simulink model "cardiac_dynamic_model"  (R2019b)
settings: Solver=FixedStepAuto  StartTime=0.0  StopTime=1  FixedStep=1e-4  RelTol=1e-3
settings Model: Creator=User  LastModifiedBy=User

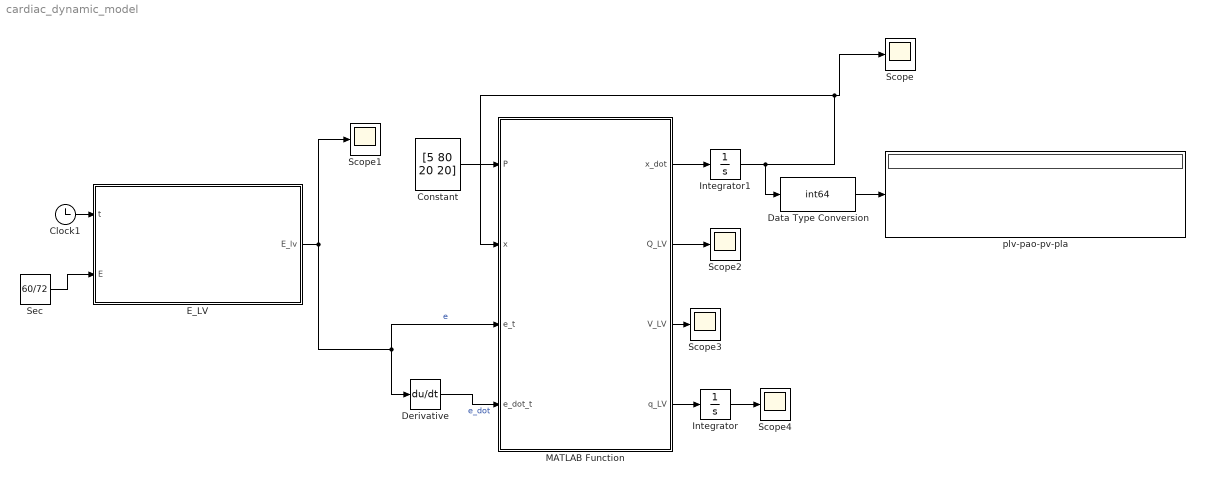
== system cardiac_dynamic_model ==
  Clock1 : Clock
  Constant : Constant  Value=[5 80 20 20]
  Data Type Conversion : DataTypeConversion  OutDataTypeStr=int64  RndMeth=Round
  Derivative : Derivative
  E_LV : Subsystem
  Integrator : Integrator
  Integrator1 : Integrator
  MATLAB Function : MATLAB Function  TreatAsAtomicUnit=on
  Scope{,1..4} (5 alike) : Scope
  Sec : Constant  Value=60/72
  plv-pao-pv-pla : Display
  wires:
  E_LV/1(E_lv) -> MATLAB Function/3(e_t), Derivative/1, Scope1/1  "e"
  Derivative/1 -> MATLAB Function/4(e_dot_t)  "e_dot"
  MATLAB Function/4(q_LV) -> Integrator/1
  MATLAB Function/2(Q_LV) -> Scope2/1
  MATLAB Function/3(V_LV) -> Scope3/1
  Integrator/1 -> Scope4/1
  Clock1/1 -> E_LV/1(t)
  Sec/1 -> E_LV/2(E)
  Integrator1/1 -> Data Type Conversion/1, MATLAB Function/2(x), Scope/1
  Data Type Conversion/1 -> plv-pao-pv-pla/1
  Constant/1 -> MATLAB Function/1(P)
  MATLAB Function/1(x_dot) -> Integrator1/1

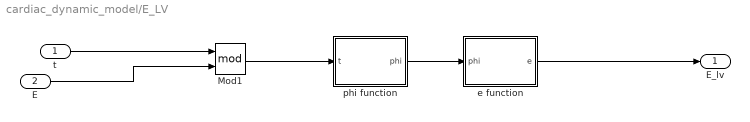
== system cardiac_dynamic_model/E_LV ==
  t : Inport
  E : Inport  Port=2
  Mod1 : Math  Operator=mod  SignedPower=off  SaturateOnIntegerOverflow=on
  e function : MATLAB Function  TreatAsAtomicUnit=on
  phi function : MATLAB Function  TreatAsAtomicUnit=on
  E_lv : Outport
  wires:
  e function/1(e) -> E_lv/1
  phi function/1(phi) -> e function/1(phi)
  Mod1/1 -> phi function/1(t)
  t/1 -> Mod1/1
  E/1 -> Mod1/2

== matlab function cardiac_dynamic_model/E_LV/phi function ==
  data: t input; phi output
function phi = fcn(t)
phi = 0.9*sin(pi/0.4*t)-0.25*sin(2*pi/0.4*t);
end

== matlab function cardiac_dynamic_model/MATLAB Function ==
  data: P input; x input; x_dot output; e_t input; e_dot_t input; Q_LV output; V_LV output; q_LV output
function [x_dot,Q_LV, V_LV, q_LV] = cardiovascular_model(P,x,e_t,e_dot_t)
Q = zeros(2,1);
p1 = 0; p2 = 0;
G1= 14.81; G2=1.46; G3=266.6; G4=20;
E_1=1/0.22;  E_2=1/20; E_3=1/1.46; E_4=1/200;
P1=5; P2=80; P3=20; P4=20;
if ((P4 - P1) > 0)
    p1 = P4 - P1;
end
    if ((P1 - P2)> 0)
        p2 = P1 - P2;
    end
    Q = [G3*p1; G2*p2];
    phase = 0;
    if Q(2,1) > 0 && Q(1,1) == 0
        phase = 1;
        G3=0;
    end
    if Q(1,1) > 0 && Q(2,1) == 0
        phase = 2;
        G2=0;
    end
    A= [e_dot_t.*4*E_4-(G3+G1) E_4/G1 0 E_4/G3;
       E_1*G2 -E_1*(G2+G1) E_1*G1 0;
     0 E_2*G1 -E_2*(G1+G4) E_2*G4;
       E_3*G3 0 E_3*G4 -E_3*(G4+G3)];
   x_dot= A*P;
   Q_LV = 0;
   if phase == 1
       Q_LV = G2*(P1 - P2);
   end 
   V_LV = 80*(1/e_t) + 10;
   q_LV = -(80 - 110)/1.46 + (15 - 80)/266.6 ;
   end

== matlab function cardiac_dynamic_model/E_LV/e function ==
  data: phi input; e output
function e = fcn(phi)
e = 0.043*(1-phi)+2.83*phi;
end
